simulink model "slrt_parker"  (R2016a)
settings: Solver=FixedStepDiscrete  StartTime=0.0  StopTime=inf  FixedStep=dts  RelTol=1e-3
InitFcn:
  | PARKER_DEPENDENCY
  | Parker_Multi_Axis_Init
  | Parker_ATI_Init
  | Parker_Home_Init
  | Parker_ScopeFormat_Init
undefined symbols (not defined in the file or in its folder): A, accel_filter_coeffs, ATI_torque_Nmm, B, counter_offset, dt, dt_ENC, dts, ENC_obs_filter_coeffs, encoder_counts, F, filter_coeffs_bias, FT_unbias_time, grav_vector, HOMING_dx, HOMING_num_joint, HOMING_tspan, HOMING_Vmov, inv_T, Kd, Kp, N_acceleration, N_bias, N_ENC_obs_filter, N_obs_velocity, N_velocity, pitch, quadrature_mode, R_FT2robot, SafetyMargin, screw_pitch, torque_constant, vel_filter_coeffs, vel_obs_filter_coeffs, Wrench_max
libraries: slrtlib x13, simulink x7, dspswit3 x6, xpcmeasurementcomputinglib x3, xpcconteclib x3, powerlib_meascontrol x2, xpcobsoletelib x1
settings Model: Creator=Roger  LastModifiedBy=arma
settings SolverCC: EnableConcurrentExecution=on
settings DataIOCC: LimitDataPoints=on  SaveFormat=Array  SignalLoggingSaveFormat=ModelDataLogs
settings OptimizationCC: BlockReduction=off  OptimizeBlockIOStorage=off  BufferReuse=off  GlobalBufferReuse=off  ExpressionFolding=off  ExpressionDepthLimit=2147483647  LocalBlockOutputs=off  InitFltsAndDblsToZero=on
settings DebuggingCC: UnderspecifiedInitializationDetection=Classic  MergeDetectMultiDrivingBlocksExec=none  SolverPrmCheckMsg=warning  MultiTaskCondExecSysMsg=warning  MultiTaskRateTransMsg=warning  FcnCallInpInsideContextMsg=EnableAllAsWarning  StateNameClashWarn=warning
settings HardwareCC: ProdBitPerPointer=32  ProdLargestAtomicFloat=None  ProdWordSize=32  ProdLongLongMode=on  ProdHWDeviceType=Generic->32-bit x86 compatible
settings ModelReferenceCC: PropagateSignalLabelsOutOfModel=off
settings SFSimCC: SimParseCustomCode=off
settings RTWCC: SystemTargetFile=slrt.tlc  TemplateMakefile=slrt_default_tmf  Description=Simulink Real-Time  RTWCompilerOptimization=on
settings SimulinkRealTimeCC: GeneratePreprocessorConditionals=Disable all  xPCisDownloadable=off  xPCisModelTimeout=off  xPCModelTimeoutSecs=15
settings ConfigComp: CovModelRefEnable=Off  CovSFcnEnable=off

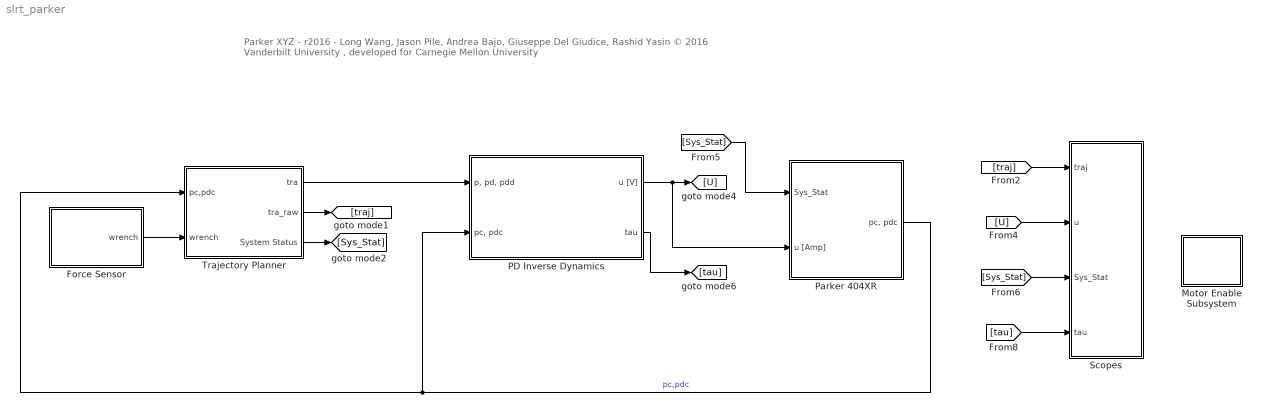
== system slrt_parker ==
  note: Parker XYZ -  r2016 - Long Wang, Jason Pile, Andrea Bajo, Giuseppe Del Giudice, Rashid Yasin
      |  © 2016 Vanderbilt University , developed for Carnegie Mellon University
  Force Sensor : Subsystem
  Motor Enable Subsystem : Subsystem
  PD Inverse Dynamics : Subsystem  TreatAsAtomicUnit=on
  Parker 404XR : Subsystem
  Scopes : Subsystem
  Trajectory Planner : Subsystem  TreatAsAtomicUnit=on
  wires:
  PD Inverse Dynamics/1(u [V]) -> Parker 404XR/2(u [Amp]), [U]
  Parker 404XR/1("pc, pdc") -> Trajectory Planner/1(pc,pdc), PD Inverse Dynamics/2("pc, pdc")  "pc,pdc"
  Trajectory Planner/1(tra) -> PD Inverse Dynamics/1("p, pd, pdd")
  Force Sensor/1(wrench) -> Trajectory Planner/2(wrench)
  [Sys_Stat] -> Parker 404XR/1(Sys_Stat)
  [traj] -> Scopes/1(traj)
  [U] -> Scopes/2(u)
  [Sys_Stat] -> Scopes/3(Sys_Stat)
  PD Inverse Dynamics/2(tau) -> [tau]
  [tau] -> Scopes/4(tau)
  Trajectory Planner/2(tra_raw) -> [traj]
  Trajectory Planner/3(System Status) -> [Sys_Stat]

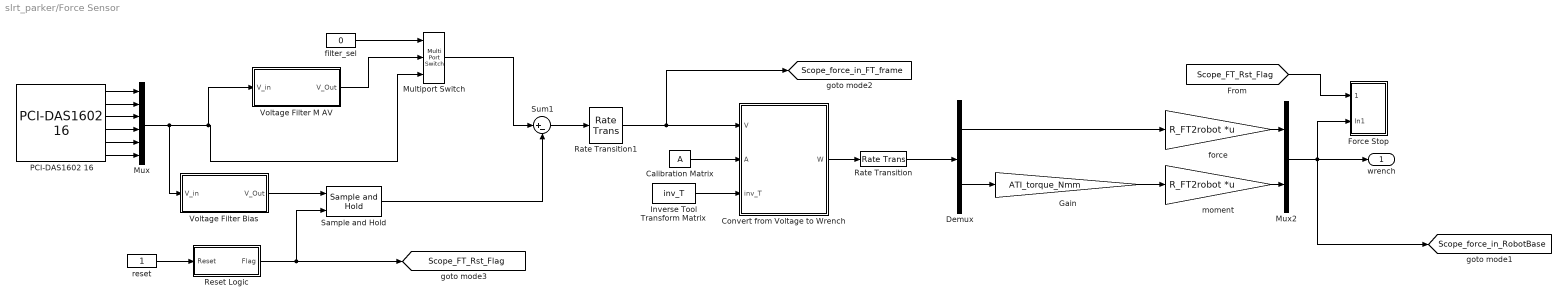
== system slrt_parker/Force Sensor ==
  Calibration Matrix : Constant  Value=A
  Convert from Voltage to Wrench : MATLAB Function  TreatAsAtomicUnit=on
  Demux : Demux  Outputs=2
  Force Stop : Subsystem
  Gain : Gain  Gain=ATI_torque_Nmm
  Inverse Tool Transform Matrix : Constant  Value=inv_T  VectorParams1D=off
  Multiport Switch : MultiPortSwitch  Inputs=2
  Mux : Mux  Inputs=6
  Mux2 : Mux  Inputs=2
  "PCI-DAS1602 16 " : xpcobsoletelib/Measurement Computing obs/A//D/PCI-DAS1602 16   channel=6  range=+-10V  mux=Differential (8 channels)  sampletime=dts  slot=-1
  Rate Transition : RateTransition  OutPortSampleTime=dt
  Rate Transition1 : RateTransition  OutPortSampleTime=dt
  Reset Logic : Subsystem
  Sample and Hold : powerlib_meascontrol/Additional Components/Sample and Hold  ic=zeros(6,1)  Ts=dts
  Sum1 : Sum  Inputs=|+-  SampleTime=dts
  Voltage Filter Bias : Subsystem
  Voltage Filter M AV : Subsystem
  filter_sel : Constant  Value=0
  force : Gain  Gain=R_FT2robot  Multiplication=Matrix(K*u)
  moment : Gain  Gain=R_FT2robot  Multiplication=Matrix(K*u)
  reset : Constant
  wrench : Outport
  tag scope: Scope_FT_Rst_Flag=global, Scope_force_in_FT_frame=global, Scope_force_in_RobotBase=global
  wires:
  "PCI-DAS1602 16 "/1 -> Mux/1
  "PCI-DAS1602 16 "/2 -> Mux/2
  "PCI-DAS1602 16 "/3 -> Mux/3
  "PCI-DAS1602 16 "/4 -> Mux/4
  "PCI-DAS1602 16 "/5 -> Mux/5
  Mux/1 -> Voltage Filter Bias/1(V_in), Voltage Filter M AV/1(V_in), Multiport Switch/3
  "PCI-DAS1602 16 "/6 -> Mux/6
  Calibration Matrix/1 -> Convert from Voltage to Wrench/2(A)
  Inverse Tool Transform Matrix/1 -> Convert from Voltage to Wrench/3(inv_T)
  Sum1/1 -> Rate Transition1/1
  Demux/1 -> force/1
  Demux/2 -> Gain/1
  force/1 -> Mux2/1
  moment/1 -> Mux2/2
  Mux2/1 -> [Scope_force_in_RobotBase], wrench/1, Force Stop/2(In1)
  Convert from Voltage to Wrench/1(W) -> Rate Transition/1
  Rate Transition/1 -> Demux/1
  Multiport Switch/1 -> Sum1/1
  filter_sel/1 -> Multiport Switch/1
  Voltage Filter Bias/1(V_Out) -> Sample and Hold/1
  Sample and Hold/1 -> Sum1/2
  reset/1 -> Reset Logic/1(Reset)
  Reset Logic/1(Flag) -> [Scope_FT_Rst_Flag], Sample and Hold/2
  Rate Transition1/1 -> [Scope_force_in_FT_frame], Convert from Voltage to Wrench/1(V)
  Voltage Filter M AV/1(V_Out) -> Multiport Switch/2
  [Scope_FT_Rst_Flag] -> Force Stop/1(ResetFlag)
  Gain/1 -> moment/1

== system slrt_parker/Motor Enable Subsystem ==
  Demux : Demux  Outputs=3
  Enable Motors : Constant  Value=ones(3,1)
  PCI-DDA08 12 to PORTA : xpcmeasurementcomputinglib/Digital Output/PCI-DDA08 12   channel=[4 5 6]  port=A  reset=[1 1 1]  initValue=[0 0 0]  chip=1  sampletime=dt  slot=-1
  wires:
  Demux/1 -> PCI-DDA08 12 to PORTA/1
  Demux/2 -> PCI-DDA08 12 to PORTA/2
  Demux/3 -> PCI-DDA08 12 to PORTA/3
  Enable Motors/1 -> Demux/1

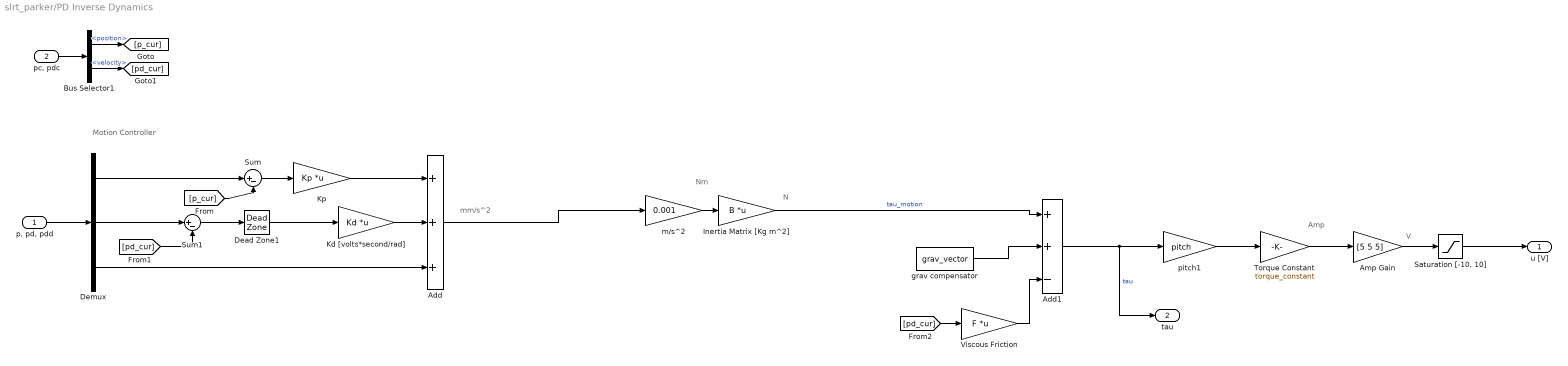
== system slrt_parker/PD Inverse Dynamics ==
  note: Motion Controller
  note: N
  note: mm/s^2
  note: Amp
  note: V
  note: Nm
  "p, pd, pdd" : Inport
  "pc, pdc" : Inport  Port=2
  Add : Sum  Inputs=+++
  Add1 : Sum  Inputs=++-  SampleTime=dt
  Amp Gain : Gain  Gain=[5 5 5]
  Bus Selector1 : BusSelector  OutputSignals=position,velocity
  Dead Zone1 : DeadZone  LowerValue=-2.5  UpperValue=2.5  SaturateOnIntegerOverflow=on
  Demux : Demux  Outputs=[3 3 3]
  Inertia Matrix [Kg m^2] : Gain  Gain=B  Multiplication=Matrix(K*u)
  Kd [volts*second/rad] : Gain  Gain=Kd  Multiplication=Matrix(K*u)
  Kp : Gain  Gain=Kp  Multiplication=Matrix(K*u)
  "Saturation [-10, 10]" : Saturate  UpperLimit=10  LowerLimit=-10
  Sum : Sum  Inputs=|+-
  Sum1 : Sum  Inputs=|+-
  Torque Constant : Gain  Gain=torque_constant
  Viscous Friction : Gain  Gain=F  Multiplication=Matrix(K*u)  SampleTime=dt
  grav compensator : Constant  Value=grav_vector
  m/s^2 : Gain  Gain=0.001
  pitch1 : Gain  Gain=pitch
  u [V] : Outport
  tau : Outport  Port=2
  wires:
  "Saturation [-10, 10]"/1 -> u [V]/1
  m/s^2/1 -> Inertia Matrix [Kg m^2]/1
  Torque Constant/1 -> Amp Gain/1
  Add1/1 -> tau/1, pitch1/1  "tau"
  pitch1/1 -> Torque Constant/1
  Amp Gain/1 -> "Saturation [-10, 10]"/1
  "p, pd, pdd"/1 -> Demux/1
  "pc, pdc"/1 -> Bus Selector1/1
  Sum/1 -> Kp/1
  Demux/1 -> Sum/1
  Demux/2 -> Sum1/1
  Bus Selector1/1 -> [p_cur]  "<position>"
  [p_cur] -> Sum/2
  [pd_cur] -> Sum1/2
  [pd_cur] -> Viscous Friction/1
  Bus Selector1/2 -> [pd_cur]  "<velocity>"
  Kp/1 -> Add/1
  Kd [volts*second/rad]/1 -> Add/2
  Demux/3 -> Add/3
  Add/1 -> m/s^2/1
  Inertia Matrix [Kg m^2]/1 -> Add1/1  "tau_motion"
  grav compensator/1 -> Add1/2
  Sum1/1 -> Dead Zone1/1
  Dead Zone1/1 -> Kd [volts*second/rad]/1
  Viscous Friction/1 -> Add1/3

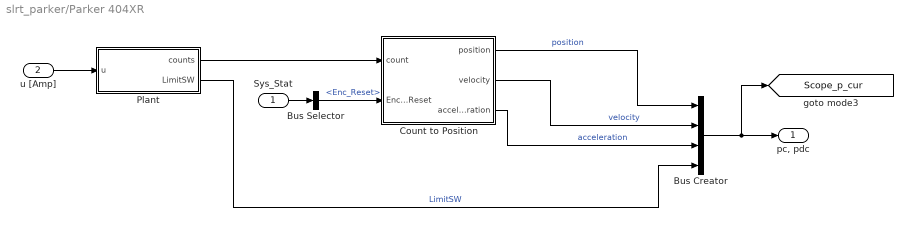
== system slrt_parker/Parker 404XR ==
  Sys_Stat : Inport
  u [Amp] : Inport  Port=2
  Bus Creator : BusCreator  Inputs=4
  Bus Selector : BusSelector  OutputSignals=Enc_Reset
  Count to Position : Subsystem
  Plant : Subsystem
  "pc, pdc" : Outport
  tag scope: Scope_p_cur=global
  wires:
  Count to Position/1(position) -> Bus Creator/1  "position"
  Plant/1(counts) -> Count to Position/1(count)
  u [Amp]/1 -> Plant/1(u)
  Bus Creator/1 -> [Scope_p_cur], "pc, pdc"/1
  Count to Position/2(velocity) -> Bus Creator/2  "velocity"
  Plant/2(LimitSW) -> Bus Creator/4  "LimitSW"
  Sys_Stat/1 -> Bus Selector/1
  Bus Selector/1 -> Count to Position/2(EncoderReset)  "<Enc_Reset>"
  Count to Position/3(acceleration) -> Bus Creator/3  "acceleration"

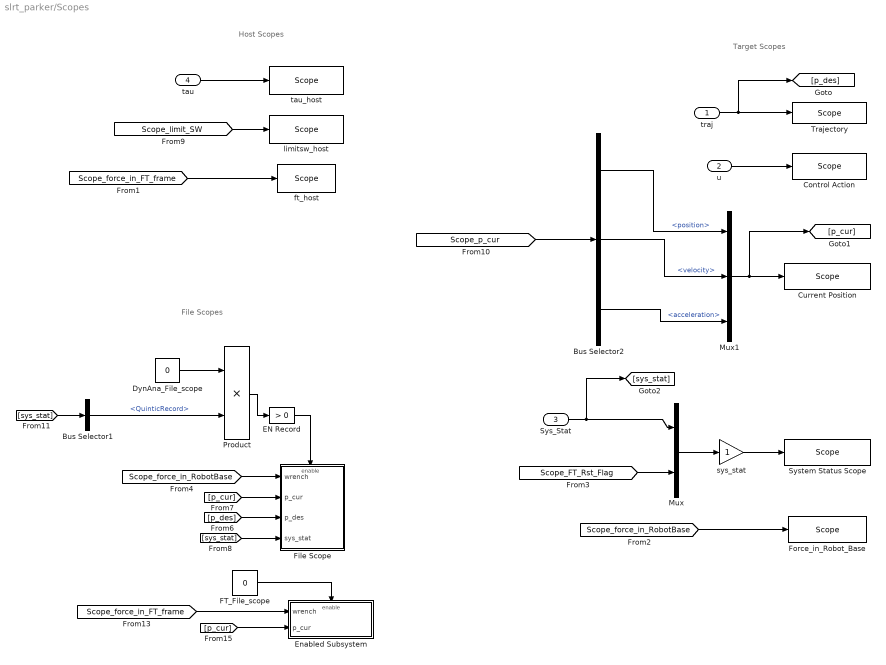
== system slrt_parker/Scopes ==
  note: Host Scopes
  note: File Scopes
  note: Target Scopes
  traj : Inport
  u : Inport  Port=2
  Sys_Stat : Inport  Port=3
  tau : Inport  Port=4
  Bus Selector1 : BusSelector  OutputSignals=QuinticRecord
  Bus Selector2 : BusSelector  OutputSignals=position,velocity,acceleration
  Control Action : slrtlib/Displays and Logging/Scope   scopeno=2  scopetype=Target  autostart=on  viewmode=Numerical  formatstr=Control_Vals_format  grid=on  ylimits=[0,0]  nosamples=Scope_Samples  noprepostsamples=0  interleave=5  triggermode=FreeRun  triggersignal=1  trigsignalfromport=off  triggerlevel=0.0  triggerslope=Either  triggerscope=1  triggersample=0  filename=data.dat  mode=Lazy  writesize=512  autorestart=off  dynamicfilemode=off  maxwritefilesize=512*1024^2
  Current Position : slrtlib/Displays and Logging/Scope   scopeno=3  scopetype=Target  autostart=on  viewmode=Numerical  formatstr=Current_Position_Vals_format  grid=on  ylimits=[0,0]  nosamples=Scope_Samples  noprepostsamples=0  interleave=1  triggermode=FreeRun  triggersignal=1  trigsignalfromport=off  triggerlevel=0.0  triggerslope=Either  triggerscope=1  triggersample=0  filename=data.dat  mode=Lazy  writesize=512  autorestart=off  dynamicfilemode=off  maxwritefilesize=512*1024^2
  DynAna_File_scope : Constant  Value=0
  EN Record : simulink/Logic and Bit Operations/Compare To Constant  relop=>  const=0  OutDataTypeStr=boolean
  Enabled Subsystem : Subsystem  TreatAsAtomicUnit=on
  FT_File_scope : Constant  Value=0
  File Scope : Subsystem
  Force_in_Robot_Base : slrtlib/Displays and Logging/Scope   scopeno=5  scopetype=Target  autostart=on  viewmode=Numerical  formatstr=forceFormat  grid=on  ylimits=[0,0]  nosamples=Scope_Samples  noprepostsamples=0  interleave=1  triggermode=FreeRun  triggersignal=1  trigsignalfromport=off  triggerlevel=0.0  triggerslope=Either  triggerscope=1  triggersample=0  filename=data.dat  mode=Lazy  writesize=512  autorestart=off  dynamicfilemode=off  maxwritefilesize=512*1024^2
  Mux : Mux  Inputs=2
  Mux1 : Mux  Inputs=3
  Product : Product  RndMeth=Zero
  System Status Scope : slrtlib/Displays and Logging/Scope   scopeno=4  scopetype=Target  autostart=on  viewmode=Numerical  formatstr=Scope_format_sys_stat  grid=on  ylimits=[0,0]  nosamples=Scope_Samples  noprepostsamples=0  interleave=1  triggermode=FreeRun  triggersignal=1  trigsignalfromport=off  triggerlevel=0.0  triggerslope=Either  triggerscope=1  triggersample=0  filename=data.dat  mode=Lazy  writesize=512  autorestart=off  dynamicfilemode=off  maxwritefilesize=512*1024^2
  Trajectory : slrtlib/Displays and Logging/Scope   scopeno=1  scopetype=Target  autostart=on  viewmode=Numerical  formatstr=p_cmd_scope_format  grid=on  ylimits=[0,0]  nosamples=25  noprepostsamples=0  interleave=1  triggermode=FreeRun  triggersignal=1  trigsignalfromport=off  triggerlevel=0.0  triggerslope=Either  triggerscope=1  triggersample=0  filename=foamdata1.dat  mode=Lazy  writesize=512  autorestart=off  dynamicfilemode=off  maxwritefilesize=512*1024^2
  ft_host : slrtlib/Displays and Logging/Scope   scopeno=12  scopetype=Host  autostart=on  viewmode=Graphical redraw  formatstr='%15.6f'  grid=on  ylimits=[0,0]  nosamples=Scope_Samples  noprepostsamples=0  interleave=1  triggermode=FreeRun  triggersignal=1  trigsignalfromport=off  triggerlevel=0.0  triggerslope=Either  triggerscope=1  triggersample=0  filename=data.dat  mode=Lazy  writesize=512  autorestart=off  dynamicfilemode=off  maxwritefilesize=512*1024^2
  limitsw_host : slrtlib/Displays and Logging/Scope   scopeno=11  scopetype=Host  autostart=on  viewmode=Graphical redraw  formatstr='%15.6f'  grid=on  ylimits=[0,0]  nosamples=Scope_Samples  noprepostsamples=0  interleave=1  triggermode=FreeRun  triggersignal=1  trigsignalfromport=off  triggerlevel=0.0  triggerslope=Either  triggerscope=1  triggersample=0  filename=data.dat  mode=Lazy  writesize=512  autorestart=off  dynamicfilemode=off  maxwritefilesize=512*1024^2
  sys_stat : Gain
  "tau_host " : slrtlib/Displays and Logging/Scope   scopeno=10  scopetype=Host  autostart=on  viewmode=Graphical redraw  formatstr='%15.6f'  grid=on  ylimits=[0,0]  nosamples=Scope_Samples  noprepostsamples=0  interleave=1  triggermode=FreeRun  triggersignal=1  trigsignalfromport=off  triggerlevel=0.0  triggerslope=Either  triggerscope=1  triggersample=0  filename=data.dat  mode=Lazy  writesize=512  autorestart=off  dynamicfilemode=off  maxwritefilesize=512*1024^2
  wires:
  [Scope_force_in_FT_frame] -> ft_host/1
  [Scope_force_in_RobotBase] -> Force_in_Robot_Base/1
  traj/1 -> [p_des], Trajectory/1
  u/1 -> Control Action/1
  [Scope_limit_SW] -> limitsw_host/1
  Sys_Stat/1 -> Mux/1, [sys_stat]
  tau/1 -> "tau_host "/1
  [Scope_FT_Rst_Flag] -> Mux/2
  Mux/1 -> sys_stat/1
  Mux1/1 -> [p_cur], Current Position/1
  [Scope_force_in_RobotBase] -> File Scope/1(wrench)
  [p_cur] -> File Scope/2(p_cur)
  [p_des] -> File Scope/3(p_des)
  [sys_stat] -> File Scope/4(sys_stat)
  [sys_stat] -> Bus Selector1/1
  EN Record/1 -> File Scope/Enable
  [Scope_p_cur] -> Bus Selector2/1
  Bus Selector2/1 -> Mux1/1  "<position>"
  Bus Selector2/2 -> Mux1/2  "<velocity>"
  Bus Selector2/3 -> Mux1/3  "<acceleration>"
  Bus Selector1/1 -> Product/2  "<QuinticRecord>"
  DynAna_File_scope/1 -> Product/1
  Product/1 -> EN Record/1
  sys_stat/1 -> System Status Scope/1
  [Scope_force_in_FT_frame] -> Enabled Subsystem/1(wrench)
  [p_cur] -> Enabled Subsystem/2(p_cur)
  FT_File_scope/1 -> Enabled Subsystem/Enable

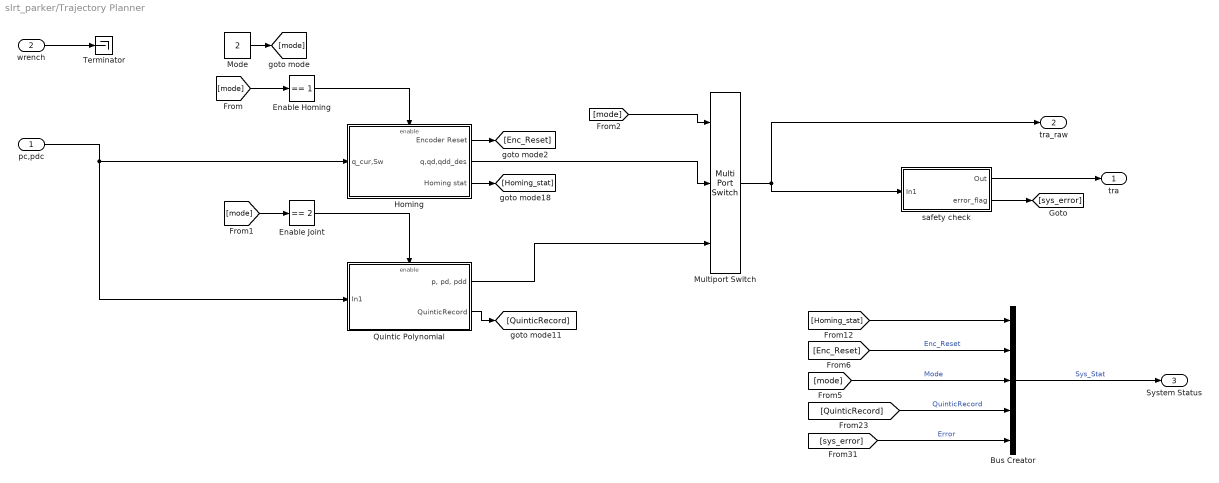
== system slrt_parker/Trajectory Planner ==
  pc,pdc : Inport
  wrench : Inport  Port=2
  Bus Creator : BusCreator  Inputs=5
  Enable Homing : simulink/Logic and Bit Operations/Compare To Constant  relop===  const=1  OutDataTypeStr=boolean
  Enable Joint : simulink/Logic and Bit Operations/Compare To Constant  relop===  const=2  OutDataTypeStr=boolean
  Homing : Subsystem
  Mode : Constant  Value=2
  Multiport Switch : MultiPortSwitch  Inputs=2
  Quintic Polynomial : Subsystem  TreatAsAtomicUnit=on
  Terminator : Terminator
  safety check : Subsystem
  tra : Outport
  tra_raw : Outport  Port=2
  System Status : Outport  Port=3
  wires:
  pc,pdc/1 -> Quintic Polynomial/1(In1), Homing/1(q_cur,Sw)
  Enable Joint/1 -> Quintic Polynomial/Enable
  Homing/2(q,qd,qdd_des) -> Multiport Switch/2
  Quintic Polynomial/1("p, pd, pdd") -> Multiport Switch/3
  Enable Homing/1 -> Homing/Enable
  Mode/1 -> [mode]
  [mode] -> Enable Homing/1
  [mode] -> Enable Joint/1
  [mode] -> Multiport Switch/1
  wrench/1 -> Terminator/1
  Homing/1(Encoder Reset) -> [Enc_Reset]
  Quintic Polynomial/2(QuinticRecord) -> [QuinticRecord]
  Homing/3(Homing stat) -> [Homing_stat]
  Multiport Switch/1 -> tra_raw/1, safety check/1(In1)
  safety check/1(Out) -> tra/1
  safety check/2(error_flag) -> [sys_error]
  Bus Creator/1 -> System Status/1  "Sys_Stat"
  [mode] -> Bus Creator/3  "Mode"
  [Enc_Reset] -> Bus Creator/2  "Enc_Reset"
  [QuinticRecord] -> Bus Creator/4  "QuinticRecord"
  [sys_error] -> Bus Creator/5  "Error"
  [Homing_stat] -> Bus Creator/1

== system slrt_parker/Force Sensor/Force Stop ==
  ResetFlag : Inport
  In1 : Inport  Port=2
  Abs : Abs
  Compare To Constant2 : simulink/Logic and Bit Operations/Compare To Constant  relop=>=  const=SafetyMargin*Wrench_max  OutDataTypeStr=boolean
  Gain : Gain
  MATLAB Function : MATLAB Function  TreatAsAtomicUnit=on
  Product : Product
  Stop Simulation : Stop
  wires:
  Abs/1 -> Gain/1
  Gain/1 -> Compare To Constant2/1
  Compare To Constant2/1 -> Stop Simulation/1
  In1/1 -> Product/1
  Product/1 -> Abs/1
  ResetFlag/1 -> MATLAB Function/1(u)
  MATLAB Function/1(y) -> Product/2

== system slrt_parker/Force Sensor/Reset Logic ==
  Reset : Inport
  Const1 : Constant
  Const2 : Constant  Value=0
  Const3 : Constant  Value=0
  N-Sample Switch : dspswit3/N-Sample Switch  N=FT_unbias_time/dts  reset=on  TriggerType=Rising edge  Ts=dts
  N-Sample Switch1 : dspswit3/N-Sample Switch  N=1  reset=off  TriggerType=Rising edge  Ts=dts
  Flag : Outport
  wires:
  Const1/1 -> N-Sample Switch/1
  N-Sample Switch/1 -> Flag/1
  Const2/1 -> N-Sample Switch/2
  Reset/1 -> N-Sample Switch1/2
  N-Sample Switch1/1 -> N-Sample Switch/3
  Const3/1 -> N-Sample Switch1/1

== system slrt_parker/Force Sensor/Voltage Filter Bias ==
  V_in : Inport  SampleTime=dts
  Discrete FIR Filter : DiscreteFir  CoefSource=Input port  SampleTime=dts  AccumDataTypeStr=Inherit: Same as product output
      settings: InputPortMap=u0,u1
  Gain : Gain  Gain=1/N_bias  SampleTime=dts
  filter_coeffs : Constant  Value=filter_coeffs_bias  SampleTime=dts
  V_Out : Outport  SampleTime=dts
  wires:
  Gain/1 -> V_Out/1
  filter_coeffs/1 -> Discrete FIR Filter/2
  Discrete FIR Filter/1 -> Gain/1
  V_in/1 -> Discrete FIR Filter/1

== system slrt_parker/Force Sensor/Voltage Filter M AV ==
  V_in : Inport  SampleTime=dts
  Discrete FIR Filter : DiscreteFir  CoefSource=Input port  SampleTime=dts  AccumDataTypeStr=Inherit: Same as product output
      settings: InputPortMap=u0,u1
  Gain : Gain  Gain=1/(dt/dts)  SampleTime=dts
  filter_coeffs : Constant  Value=ones(dt/dts,1)  SampleTime=dts
  V_Out : Outport  SampleTime=dts
  wires:
  V_in/1 -> Discrete FIR Filter/1
  Discrete FIR Filter/1 -> Gain/1
  filter_coeffs/1 -> Discrete FIR Filter/2
  Gain/1 -> V_Out/1

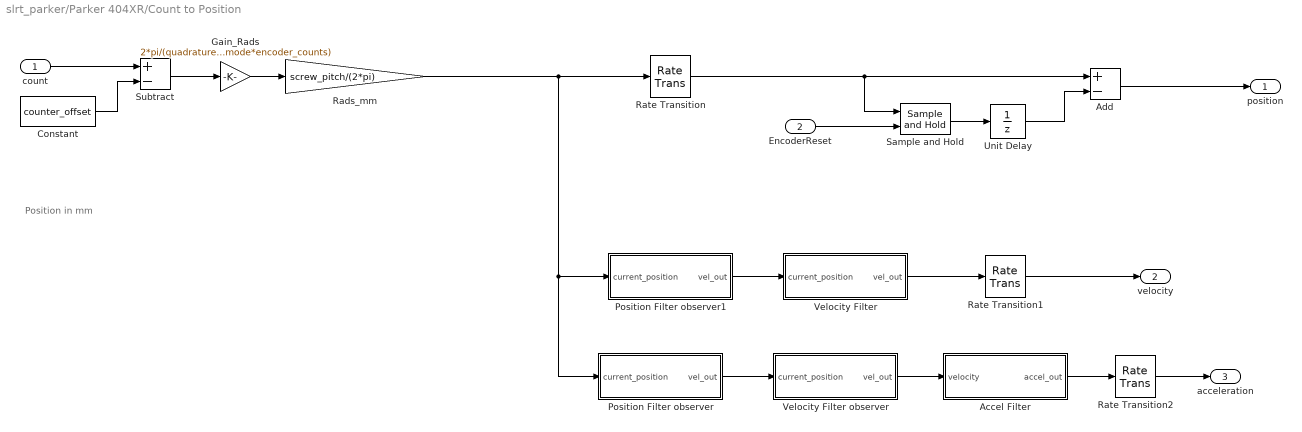
== system slrt_parker/Parker 404XR/Count to Position ==
  note: Position in mm
  count : Inport
  EncoderReset : Inport  Port=2
  Accel Filter : Subsystem
  Add : Sum  Inputs=+-
  Constant : Constant  Value=counter_offset
  Gain_Rads : Gain  Gain=2*pi/(quadrature_mode*encoder_counts)
  Position Filter observer : Subsystem
  Position Filter observer1 : Subsystem
  Rads_mm : Gain  Gain=screw_pitch/(2*pi)
  Rate Transition : RateTransition  OutPortSampleTime=dt
  Rate Transition1 : RateTransition  OutPortSampleTime=dt
  Rate Transition2 : RateTransition  OutPortSampleTime=dt
  Sample and Hold : powerlib_meascontrol/Additional Components/Sample and Hold  ic=zeros(3,1)  Ts=dt
  Subtract : Sum  Inputs=+-
  Unit Delay : UnitDelay  SampleTime=-1
  Velocity Filter : Subsystem
  Velocity Filter observer : Subsystem
  position : Outport
  velocity : Outport  Port=2
  acceleration : Outport  Port=3
  wires:
  Constant/1 -> Subtract/2
  count/1 -> Subtract/1
  Subtract/1 -> Gain_Rads/1
  Gain_Rads/1 -> Rads_mm/1
  Add/1 -> position/1
  Rads_mm/1 -> Rate Transition/1, Position Filter observer1/1(current_position), Position Filter observer/1(current_position)
  Velocity Filter/1(vel_out) -> Rate Transition1/1
  Accel Filter/1(accel_out) -> Rate Transition2/1
  Velocity Filter observer/1(vel_out) -> Accel Filter/1(velocity)
  Position Filter observer/1(vel_out) -> Velocity Filter observer/1(current_position)
  Position Filter observer1/1(vel_out) -> Velocity Filter/1(current_position)
  Sample and Hold/1 -> Unit Delay/1
  Rate Transition/1 -> Sample and Hold/1, Add/1
  Rate Transition1/1 -> velocity/1
  Rate Transition2/1 -> acceleration/1
  EncoderReset/1 -> Sample and Hold/2
  Unit Delay/1 -> Add/2

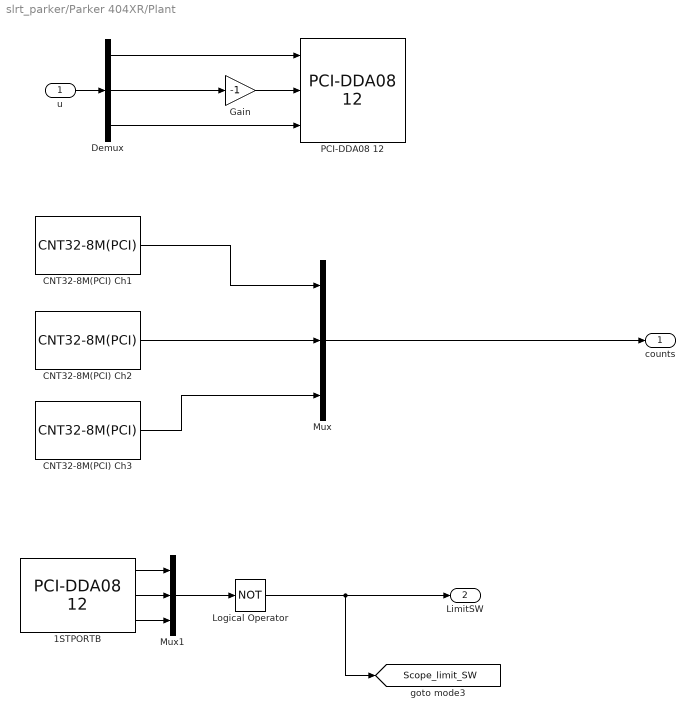
== system slrt_parker/Parker 404XR/Plant ==
  u : Inport
  "1STPORTB " : xpcmeasurementcomputinglib/Digital Input/PCI-DDA08 12   channel=[3 4 7]  port=C  chip=1  sampletime=dt  slot=-1
  CNT32-8M(PCI) Ch1 : xpcconteclib/Incremental Encoder/CNT32-8M(PCI)   Channel=1  OperationMode=2-phase Input Synchronous Clear Multiply by 4  DigitalFilter=No filtering  PulseInput=Differential line receiver input  Direction=Down in the clockwise direction/Up in the counterclockwise direction  InitialValue=counter_offset  LoadInitialValue=on  SampleTime=dt_ENC  PciSlot=-1  StartMethod=Model Start  StopMethod=Model Terminate  ZeroClearRising=off  ZeroClearFalling=off  ZeroClearMatch0=off  ZeroClearMatch1=off  PresetRising=off  PresetFalling=off  PresetMatch0=off  PresetMatch1=off  PresetValue=0  Match0Value=0  Match1Value=0  OutputSignalMatch0=off  OutputSignalMatch1=off  OutputSignalAbnormal=off  OutputSignalDigitalFilter=off  OutputSignalAlarm=off  OneShotDuration=10 microseconds  IndexEnable=Disable  IndexLogic=Positive (Active High)  EnableDigitalInput=off  EnableDigitalOutput=off  DigitalOutputInitialValue=None  DigitalOutputFinalValue=None
  CNT32-8M(PCI) Ch2 : xpcconteclib/Incremental Encoder/CNT32-8M(PCI)   Channel=2  OperationMode=2-phase Input Synchronous Clear Multiply by 4  DigitalFilter=No filtering  PulseInput=Differential line receiver input  Direction=Up in the clockwise direction/Down in the counterclockwise direction  InitialValue=counter_offset  LoadInitialValue=on  SampleTime=dt_ENC  PciSlot=-1  StartMethod=Model Start  StopMethod=Model Terminate  ZeroClearRising=off  ZeroClearFalling=off  ZeroClearMatch0=off  ZeroClearMatch1=off  PresetRising=off  PresetFalling=off  PresetMatch0=off  PresetMatch1=off  PresetValue=0  Match0Value=0  Match1Value=0  OutputSignalMatch0=off  OutputSignalMatch1=off  OutputSignalAbnormal=off  OutputSignalDigitalFilter=off  OutputSignalAlarm=off  OneShotDuration=10 microseconds  IndexEnable=Disable  IndexLogic=Positive (Active High)  EnableDigitalInput=off  EnableDigitalOutput=off  DigitalOutputInitialValue=None  DigitalOutputFinalValue=None
  CNT32-8M(PCI) Ch3 : xpcconteclib/Incremental Encoder/CNT32-8M(PCI)   Channel=3  OperationMode=2-phase Input Synchronous Clear Multiply by 4  DigitalFilter=No filtering  PulseInput=Differential line receiver input  Direction=Down in the clockwise direction/Up in the counterclockwise direction  InitialValue=counter_offset  LoadInitialValue=on  SampleTime=dt_ENC  PciSlot=-1  StartMethod=Model Start  StopMethod=Model Terminate  ZeroClearRising=off  ZeroClearFalling=off  ZeroClearMatch0=off  ZeroClearMatch1=off  PresetRising=off  PresetFalling=off  PresetMatch0=off  PresetMatch1=off  PresetValue=0  Match0Value=0  Match1Value=0  OutputSignalMatch0=off  OutputSignalMatch1=off  OutputSignalAbnormal=off  OutputSignalDigitalFilter=off  OutputSignalAlarm=off  OneShotDuration=10 microseconds  IndexEnable=Disable  IndexLogic=Positive (Active High)  EnableDigitalInput=off  EnableDigitalOutput=off  DigitalOutputInitialValue=None  DigitalOutputFinalValue=None
  Demux : Demux  Outputs=3
  Gain : Gain  Gain=-1
  Logical Operator : Logic  Operator=NOT  Inputs=1  AllPortsSameDT=off  OutDataTypeStr=boolean
  Mux : Mux  Inputs=3
  Mux1 : Mux  Inputs=3
  "PCI-DDA08 12 " : xpcmeasurementcomputinglib/D//A/PCI-DDA08 12   channel=[4 5 6]  range=[-10 -10 -10]  reset=[1 1 1]  initValue=[0 0 0]  sampletime=dt  pci_dev=-1
  counts : Outport
  LimitSW : Outport  Port=2
  tag scope: Scope_limit_SW=global
  wires:
  Demux/3 -> "PCI-DDA08 12 "/3
  Gain/1 -> "PCI-DDA08 12 "/2
  CNT32-8M(PCI) Ch3/1 -> Mux/3
  CNT32-8M(PCI) Ch2/1 -> Mux/2
  CNT32-8M(PCI) Ch1/1 -> Mux/1
  Demux/2 -> Gain/1
  Demux/1 -> "PCI-DDA08 12 "/1
  u/1 -> Demux/1
  "1STPORTB "/1 -> Mux1/1
  "1STPORTB "/2 -> Mux1/2
  "1STPORTB "/3 -> Mux1/3
  Mux/1 -> counts/1
  Mux1/1 -> Logical Operator/1
  Logical Operator/1 -> [Scope_limit_SW], LimitSW/1

== system slrt_parker/Scopes/Enabled Subsystem ==
  wrench : Inport
  p_cur : Inport  Port=2
  Enable : EnablePort
  Gain : Gain
  Gain1 : Gain
  "ft_Scope " : slrtlib/Displays and Logging/Scope   scopeno=23  scopetype=File  autostart=on  viewmode=Graphical redraw  formatstr='%15.6f'  grid=on  ylimits=[0,0]  nosamples=50000  noprepostsamples=0  interleave=1  triggermode=FreeRun  triggersignal=1  trigsignalfromport=off  triggerlevel=0.0  triggerslope=Either  triggerscope=1  triggersample=0  filename=Ft_<%%%>.dat  mode=Lazy  writesize=512  autorestart=on  dynamicfilemode=on  maxwritefilesize=512*1024^2
  "pc_Scope " : slrtlib/Displays and Logging/Scope   scopeno=24  scopetype=File  autostart=on  viewmode=Graphical redraw  formatstr='%15.6f'  grid=on  ylimits=[0,0]  nosamples=50000  noprepostsamples=0  interleave=1  triggermode=FreeRun  triggersignal=1  trigsignalfromport=off  triggerlevel=0.0  triggerslope=Either  triggerscope=1  triggersample=0  filename=Pc_<%%%>.dat  mode=Lazy  writesize=512  autorestart=on  dynamicfilemode=on  maxwritefilesize=512*1024^2
  wires:
  wrench/1 -> Gain1/1
  p_cur/1 -> Gain/1
  Gain/1 -> "pc_Scope "/1
  Gain1/1 -> "ft_Scope "/1

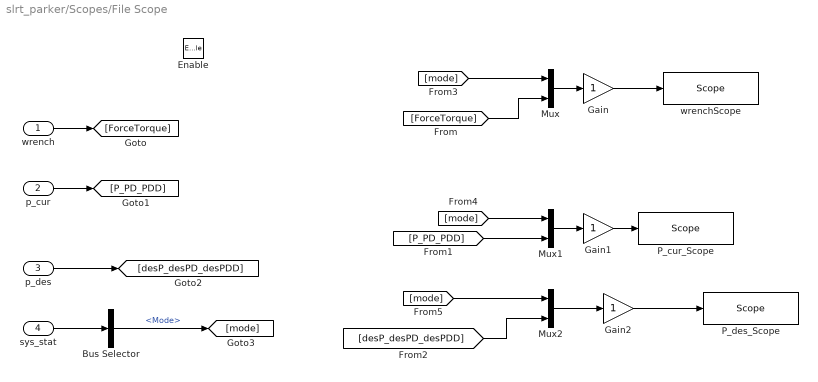
== system slrt_parker/Scopes/File Scope ==
  wrench : Inport
  p_cur : Inport  Port=2
  p_des : Inport  Port=3
  sys_stat : Inport  Port=4
  Enable : EnablePort
  Bus Selector : BusSelector  OutputSignals=Mode
  Gain : Gain
  Gain1 : Gain
  Gain2 : Gain
  Mux : Mux  Inputs=2
  Mux1 : Mux  Inputs=2
  Mux2 : Mux  Inputs=2
  P_cur_Scope : slrtlib/Displays and Logging/Scope   scopeno=21  scopetype=File  autostart=on  viewmode=Numerical  formatstr=forceFormat  grid=on  ylimits=[0,0]  nosamples=50000  noprepostsamples=0  interleave=1  triggermode=FreeRun  triggersignal=1  trigsignalfromport=off  triggerlevel=0.0  triggerslope=Either  triggerscope=1  triggersample=0  filename=Cur_<%%%>.dat  mode=Lazy  writesize=512  autorestart=on  dynamicfilemode=on  maxwritefilesize=512*1024^2
  P_des_Scope : slrtlib/Displays and Logging/Scope   scopeno=22  scopetype=File  autostart=on  viewmode=Numerical  formatstr=forceFormat  grid=on  ylimits=[0,0]  nosamples=50000  noprepostsamples=0  interleave=1  triggermode=FreeRun  triggersignal=1  trigsignalfromport=off  triggerlevel=0.0  triggerslope=Either  triggerscope=1  triggersample=0  filename=Des_<%%%>.dat  mode=Lazy  writesize=512  autorestart=on  dynamicfilemode=on  maxwritefilesize=512*1024^2
  wrenchScope : slrtlib/Displays and Logging/Scope   scopeno=20  scopetype=File  autostart=on  viewmode=Numerical  formatstr=forceFormat  grid=on  ylimits=[0,0]  nosamples=50000  noprepostsamples=0  interleave=1  triggermode=FreeRun  triggersignal=1  trigsignalfromport=off  triggerlevel=0.0  triggerslope=Either  triggerscope=1  triggersample=0  filename=We_<%%%>.dat  mode=Lazy  writesize=512  autorestart=on  dynamicfilemode=on  maxwritefilesize=512*1024^2
  wires:
  wrench/1 -> [ForceTorque]
  p_cur/1 -> [P_PD_PDD]
  p_des/1 -> [desP_desPD_desPDD]
  sys_stat/1 -> Bus Selector/1
  Bus Selector/1 -> [mode]  "<Mode>"
  Mux/1 -> Gain/1
  [ForceTorque] -> Mux/2
  [mode] -> Mux/1
  Mux1/1 -> Gain1/1
  [mode] -> Mux1/1
  [P_PD_PDD] -> Mux1/2
  Mux2/1 -> Gain2/1
  [mode] -> Mux2/1
  [desP_desPD_desPDD] -> Mux2/2
  Gain/1 -> wrenchScope/1
  Gain1/1 -> P_cur_Scope/1
  Gain2/1 -> P_des_Scope/1

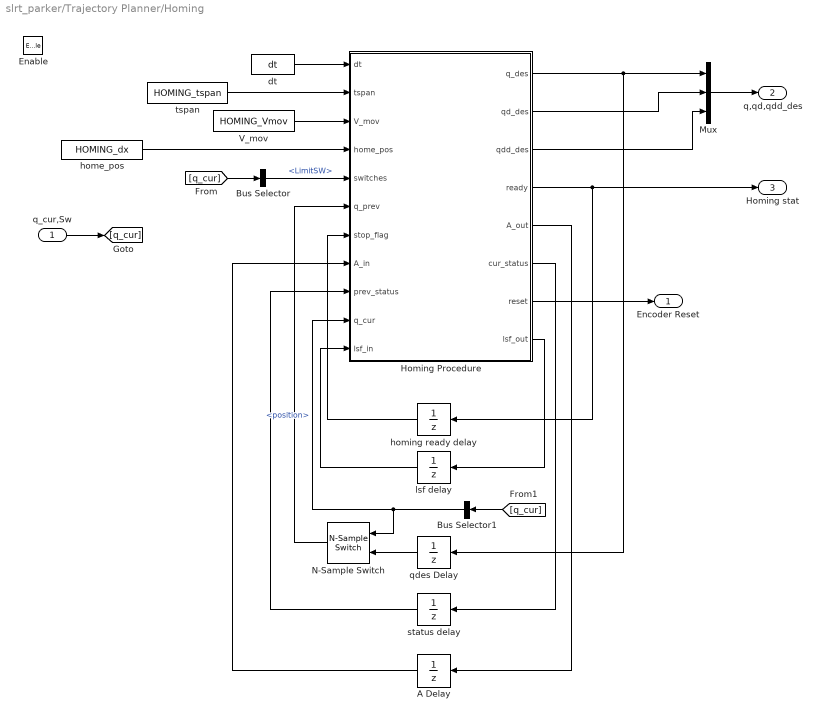
== system slrt_parker/Trajectory Planner/Homing ==
  q_cur,Sw : Inport
  Enable : EnablePort  StatesWhenEnabling=reset
  A Delay : UnitDelay  InitialCondition=zeros(HOMING_num_joint,4)  SampleTime=dt
  Bus Selector : BusSelector  OutputSignals=LimitSW
  Bus Selector1 : BusSelector  OutputSignals=position
  Homing Procedure : MATLAB Function  TreatAsAtomicUnit=on
  Mux : Mux  Inputs=3
  N-Sample Switch : dspswit3/N-Sample Switch  N=1  reset=off  TriggerType=Rising edge  Ts=dt
  V_mov : Constant  Value=HOMING_Vmov  SampleTime=dt
  dt : Constant  Value=dt  SampleTime=dt
  home_pos : Constant  Value=HOMING_dx  SampleTime=dt
  homing ready delay : UnitDelay  SampleTime=dt
  lsf delay : UnitDelay  InitialCondition=ones(HOMING_num_joint,1)  SampleTime=dt
  qdes Delay : UnitDelay  InitialCondition=zeros(HOMING_num_joint,1)  SampleTime=dt
  status delay : UnitDelay  SampleTime=dt
  tspan : Constant  Value=HOMING_tspan  SampleTime=dt
  Encoder Reset : Outport
  q,qd,qdd_des : Outport  Port=2
  Homing stat : Outport  Port=3
  wires:
  Homing Procedure/1(q_des) -> qdes Delay/1, Mux/1
  Bus Selector/1 -> Homing Procedure/5(switches)  "<LimitSW>"
  Homing Procedure/4(ready) -> homing ready delay/1, Homing stat/1
  homing ready delay/1 -> Homing Procedure/7(stop_flag)
  dt/1 -> Homing Procedure/1(dt)
  qdes Delay/1 -> N-Sample Switch/2
  N-Sample Switch/1 -> Homing Procedure/6(q_prev)
  Bus Selector1/1 -> Homing Procedure/10(q_cur), N-Sample Switch/1  "<position>"
  home_pos/1 -> Homing Procedure/4(home_pos)
  Homing Procedure/5(A_out) -> A Delay/1
  A Delay/1 -> Homing Procedure/8(A_in)
  Homing Procedure/6(cur_status) -> status delay/1
  status delay/1 -> Homing Procedure/9(prev_status)
  Homing Procedure/7(reset) -> Encoder Reset/1
  Homing Procedure/8(lsf_out) -> lsf delay/1
  lsf delay/1 -> Homing Procedure/11(lsf_in)
  Homing Procedure/2(qd_des) -> Mux/2
  Homing Procedure/3(qdd_des) -> Mux/3
  Mux/1 -> q,qd,qdd_des/1
  q_cur,Sw/1 -> [q_cur]
  [q_cur] -> Bus Selector/1
  [q_cur] -> Bus Selector1/1
  tspan/1 -> Homing Procedure/2(tspan)
  V_mov/1 -> Homing Procedure/3(V_mov)

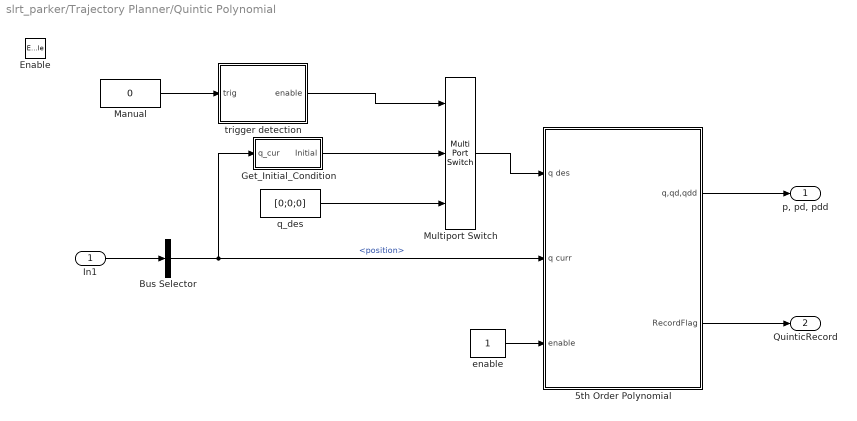
== system slrt_parker/Trajectory Planner/Quintic Polynomial ==
  In1 : Inport
  Enable : EnablePort  StatesWhenEnabling=reset
  5th Order Polynomial : Subsystem
  Bus Selector : BusSelector  OutputSignals=position
  Get_Initial_Condition : Subsystem
  Manual : Constant  Value=0
  Multiport Switch : MultiPortSwitch  DataPortOrder=Zero-based contiguous  Inputs=2
  enable : Constant
  q_des : Constant  Value=[0;0;0]
  trigger detection : Subsystem
  "p, pd, pdd" : Outport  InitialOutput=zeros(9,1)
  QuinticRecord : Outport  Port=2  InitialOutput=0
  wires:
  enable/1 -> 5th Order Polynomial/3(enable)
  In1/1 -> Bus Selector/1
  Bus Selector/1 -> 5th Order Polynomial/2(q curr), Get_Initial_Condition/1(q_cur)  "<position>"
  5th Order Polynomial/1(q,qd,qdd) -> "p, pd, pdd"/1
  Multiport Switch/1 -> 5th Order Polynomial/1(q des)
  q_des/1 -> Multiport Switch/3
  Get_Initial_Condition/1(Initial) -> Multiport Switch/2
  5th Order Polynomial/2(RecordFlag) -> QuinticRecord/1
  Manual/1 -> trigger detection/1(trig)
  trigger detection/1(enable) -> Multiport Switch/1

== system slrt_parker/Trajectory Planner/safety check ==
  In1 : Inport
  Unit Delay2 : UnitDelay  InitialCondition=zeros(9,1)  SampleTime=-1
  Unit Delay3 : UnitDelay  SampleTime=-1
  false detection : MATLAB Function  TreatAsAtomicUnit=on
  Out : Outport
  error_flag : Outport  Port=2
  wires:
  false detection/1(pva_allowed) -> Unit Delay2/1, Out/1
  Unit Delay2/1 -> false detection/2(pva_prev)
  In1/1 -> false detection/1(pva_cmd)
  Unit Delay3/1 -> false detection/3(error_prev)
  false detection/2(error_flag) -> Unit Delay3/1, error_flag/1

== system slrt_parker/Parker 404XR/Count to Position/Accel Filter ==
  note: current velocity
  velocity : Inport
  Discrete Derivative1 : simulink/Discrete/Discrete Derivative  gainval=1.0  ICPrevScaledInput=0.0  InputProcessing=Inherited  OutMin=[]  OutMax=[]  OutDataType=sfix(16)  OutScaling=2^-10  DoSatur=off
  Discrete FIR Filter : DiscreteFir  CoefSource=Input port  AccumDataTypeStr=Inherit: Same as product output
      settings: InputPortMap=u0,u1
  Gain : Gain  Gain=1/N_acceleration
  vel_filter_coeffs : Constant  Value=accel_filter_coeffs
  accel_out : Outport
  wires:
  Discrete FIR Filter/1 -> Gain/1
  vel_filter_coeffs/1 -> Discrete FIR Filter/2
  Gain/1 -> accel_out/1
  velocity/1 -> Discrete Derivative1/1
  Discrete Derivative1/1 -> Discrete FIR Filter/1

== system slrt_parker/Parker 404XR/Count to Position/Position Filter observer ==
  note: current velocity
  current_position : Inport
  Discrete FIR Filter : DiscreteFir  CoefSource=Input port  AccumDataTypeStr=Inherit: Same as product output
      settings: InputPortMap=u0,u1
  Gain : Gain  Gain=1/N_ENC_obs_filter
  encoder obsever filter : Constant  Value=ENC_obs_filter_coeffs
  vel_out : Outport
  wires:
  current_position/1 -> Discrete FIR Filter/1
  Gain/1 -> vel_out/1
  encoder obsever filter/1 -> Discrete FIR Filter/2
  Discrete FIR Filter/1 -> Gain/1

== system slrt_parker/Parker 404XR/Count to Position/Position Filter observer1 ==
  note: current velocity
  current_position : Inport
  Discrete FIR Filter : DiscreteFir  CoefSource=Input port  AccumDataTypeStr=Inherit: Same as product output
      settings: InputPortMap=u0,u1
  Gain : Gain  Gain=1/N_ENC_obs_filter
  encoder obsever filter : Constant  Value=ENC_obs_filter_coeffs
  vel_out : Outport
  wires:
  Discrete FIR Filter/1 -> Gain/1
  encoder obsever filter/1 -> Discrete FIR Filter/2
  Gain/1 -> vel_out/1
  current_position/1 -> Discrete FIR Filter/1

== system slrt_parker/Parker 404XR/Count to Position/Velocity Filter ==
  note: current velocity
  current_position : Inport
  Discrete Derivative : simulink/Discrete/Discrete Derivative  gainval=1.0  ICPrevScaledInput=0.0  InputProcessing=Inherited  OutMin=[]  OutMax=[]  OutDataType=sfix(16)  OutScaling=2^-10  DoSatur=off
  Discrete FIR Filter : DiscreteFir  CoefSource=Input port  AccumDataTypeStr=Inherit: Same as product output
      settings: InputPortMap=u0,u1
  Gain : Gain  Gain=1/N_velocity
  vel_filter_coeffs : Constant  Value=vel_filter_coeffs
  vel_out : Outport
  wires:
  current_position/1 -> Discrete Derivative/1
  Discrete Derivative/1 -> Discrete FIR Filter/1
  Gain/1 -> vel_out/1
  vel_filter_coeffs/1 -> Discrete FIR Filter/2
  Discrete FIR Filter/1 -> Gain/1

== system slrt_parker/Parker 404XR/Count to Position/Velocity Filter observer ==
  note: current velocity
  current_position : Inport
  Discrete Derivative : simulink/Discrete/Discrete Derivative  gainval=1.0  ICPrevScaledInput=0.0  InputProcessing=Inherited  OutMin=[]  OutMax=[]  OutDataType=sfix(16)  OutScaling=2^-10  DoSatur=off
  Discrete FIR Filter : DiscreteFir  CoefSource=Input port  AccumDataTypeStr=Inherit: Same as product output
      settings: InputPortMap=u0,u1
  Gain : Gain  Gain=1/N_obs_velocity
  vel_filter_coeffs : Constant  Value=vel_obs_filter_coeffs
  vel_out : Outport
  wires:
  Discrete FIR Filter/1 -> Gain/1
  vel_filter_coeffs/1 -> Discrete FIR Filter/2
  Gain/1 -> vel_out/1
  Discrete Derivative/1 -> Discrete FIR Filter/1
  current_position/1 -> Discrete Derivative/1

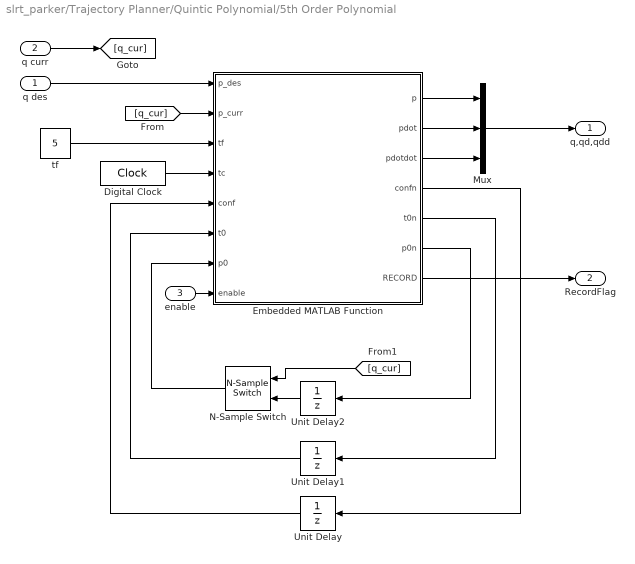
== system slrt_parker/Trajectory Planner/Quintic Polynomial/5th Order Polynomial ==
  q des : Inport
  q curr : Inport  Port=2
  enable : Inport  Port=3
  Digital Clock : DigitalClock  SampleTime=dt
  Embedded MATLAB Function : MATLAB Function  TreatAsAtomicUnit=on
  Mux : Mux  Inputs=3
  N-Sample Switch : dspswit3/N-Sample Switch  N=1  reset=off  TriggerType=Rising edge  Ts=dt
  Unit Delay : UnitDelay  SampleTime=dt
  Unit Delay1 : UnitDelay  SampleTime=dt
  Unit Delay2 : UnitDelay  SampleTime=dt
  tf : Constant  Value=5  SampleTime=dt
  q,qd,qdd : Outport
  RecordFlag : Outport  Port=2
  wires:
  Embedded MATLAB Function/4(confn) -> Unit Delay/1
  Unit Delay/1 -> Embedded MATLAB Function/5(conf)
  Embedded MATLAB Function/5(t0n) -> Unit Delay1/1
  Embedded MATLAB Function/6(p0n) -> Unit Delay2/1
  Unit Delay1/1 -> Embedded MATLAB Function/6(t0)
  Digital Clock/1 -> Embedded MATLAB Function/4(tc)
  q des/1 -> Embedded MATLAB Function/1(p_des)
  tf/1 -> Embedded MATLAB Function/3(tf)
  enable/1 -> Embedded MATLAB Function/8(enable)
  Embedded MATLAB Function/1(p) -> Mux/1
  Embedded MATLAB Function/2(pdot) -> Mux/2
  Mux/1 -> q,qd,qdd/1
  Embedded MATLAB Function/3(pdotdot) -> Mux/3
  N-Sample Switch/1 -> Embedded MATLAB Function/7(p0)
  Unit Delay2/1 -> N-Sample Switch/2
  q curr/1 -> [q_cur]
  [q_cur] -> Embedded MATLAB Function/2(p_curr)
  [q_cur] -> N-Sample Switch/1
  Embedded MATLAB Function/7(RECORD) -> RecordFlag/1

== system slrt_parker/Trajectory Planner/Quintic Polynomial/Get_Initial_Condition ==
  q_cur : Inport
  N-Sample Switch : dspswit3/N-Sample Switch  N=1  reset=off  TriggerType=Rising edge  Ts=dt
  Unit Delay : UnitDelay  InitialCondition=zeros(3,1)  SampleTime=-1
  Initial : Outport
  wires:
  N-Sample Switch/1 -> Unit Delay/1, Initial/1
  Unit Delay/1 -> N-Sample Switch/2
  q_cur/1 -> N-Sample Switch/1

== system slrt_parker/Trajectory Planner/Quintic Polynomial/trigger detection ==
  trig : Inport
  Counter : dspswit3/Counter  Direction=Up  CountEvent=Rising edge  CounterSize=User defined  MaxCount=255  InitialCount=0  Output=Count  HitValue=32  ResetInput=off  SamplesPerFrame=1  Ts=1  CntDtype=double  HitDtype=Boolean
  MATLAB Function : MATLAB Function  TreatAsAtomicUnit=on
  Unit Delay : UnitDelay  SampleTime=dt
  enable : Outport
  wires:
  MATLAB Function/1(enable) -> enable/1, Unit Delay/1
  Counter/1 -> MATLAB Function/1(trig)
  Unit Delay/1 -> MATLAB Function/2(trig_history)
  trig/1 -> Counter/1

== matlab function slrt_parker/Trajectory Planner/Homing/Homing Procedure ==
  data: dt input; tspan input; V_mov input; home_pos input; switches input; q_prev input; q_des output; qd_des output; qdd_des output; ready output; stop_flag input; A_in input; prev_status input; A_out output; cur_status output; reset output; q_cur input; lsf_in input; lsf_out output
% this function executes a homing sequence for the parallel robots
% status definition:
%       1: keep homing
%       0: stop homing
% stop flag definition:
%       0: all limit switches have not been reached
%       1: limit switches reached, calculate trajectory to home config
%       2: run 5th order poly
%       3: home complete - reset and hold position
%       4: turn off reset, hold at 0

function [q_des,qd_des,qdd_des,ready,A_out,cur_status,reset,lsf_out] = homing(dt,tspan,V_mov,home_pos,switches,q_prev,stop_flag,A_in,prev_status,q_cur,lsf_in)
% V_mov=5; % leg velocity while homing (mm/s)
% tspan=10;    % time to execute path plan (sec)
N=length(q_prev);
qd_des=zeros(N,1); % default desired velocity
qdd_des=zeros(N,1); %default desired acceleration

% read limit switches
% when limit switches are reached, switch=1
status=ones(N,1)-switches;    % update triggered switches
lsf_out=lsf_in.*status;
if stop_flag==1
    dx=home_pos;    % total displacement
    A_out=zeros(N,4);   % allocate memory for coefficients

    % construct coefficients
    for i=1:N
        A_out(i,:)=[q_prev(i),10*dx(i), -15*dx(i), 6*dx(i)];
    end
    cur_status=1;
    cur_t=cur_status*dt/tspan;
    T=[1;cur_t^3;cur_t^4;cur_t^5];    % exponential time vector
    q_des=A_out*T;  % current desired position 
    ready=2;        % continue with path plan (should be 2)
    reset=0;
elseif stop_flag==2
    
    if prev_status>=(tspan/dt)    % reached position goal
        T=[1;1;1;1];
        q_des=A_in*T;
        cur_status=prev_status;
        A_out=[q_des,zeros(N,3)];
        ready=3;
        reset=0;
    else    % continue on the trajectory
        cur_t=prev_status*dt/tspan; % current normalized time [0 -> 1]
        T=[1;cur_t^3;cur_t^4;cur_t^5];    % exponential time vector
        q_des=A_in*T;  % current desired position
        cur_status=prev_status+1; % update status step
        A_out=A_in; % maintain current coefficients  
        ready=2;
        reset=0;
    end
elseif stop_flag==3
    cur_status=0;
    A_out=zeros(N,4);
    q_des=q_cur;
    ready=4;
    reset=1;
elseif stop_flag==4
    cur_status=0;
    A_out=zeros(N,4);
    q_des=q_cur*0;
    ready=4;
    reset=0;
else
    % check homing status    
    if (sum(lsf_out))==0   % all limit switches have been reached
        q_des=q_prev;       % stop motion
        ready=1;            % homing finished
        cur_status=0;
        A_out=zeros(N,4);
        reset=0;
    else    % continue homing
        q_des=q_prev + status.*V_mov*dt;   % move legs that have not reached goal
        ready=0;            % homing not finished
        cur_status=0;
        A_out=zeros(N,4);
        reset=0;
    end
end

== matlab function slrt_parker/Force Sensor/Convert from Voltage to Wrench ==
  data: V input; W output; A input; inv_T input
function W = Convert_Function(V,A,inv_T)%A_vec,p)

W = inv_T*A*V;

== matlab function slrt_parker/Trajectory Planner/Quintic Polynomial/trigger detection/MATLAB Function ==
  data: trig input; enable output; trig_history input
function enable= fcn(trig,trig_history)
%#codegen
%%  This func is just to detect a rising trigger
%   Once this rising trigger detected, this manual enable will be locked
%   until mode change
if trig_history==0
    if trig==0
        enable=0;
    else
        enable=1;
    end
else
    enable = 1;
end

== matlab function slrt_parker/Trajectory Planner/Quintic Polynomial/5th Order Polynomial/Embedded MATLAB Function ==
  data: p output; p_des input; p_curr input; tf input; tc input; pdot output; pdotdot output; conf input; confn output; t0 input; t0n output; p0n output; p0 input; enable input; RECORD output
function [p,pdot,pdotdot,confn,t0n,p0n,RECORD] = fifth_order_p(p_des,p_curr,tf,tc,conf,t0,p0,enable)

n = 3;
RECORD = 0;

if enable == 0                  % Configuration space is not used (pdot = 0). 
    p = p_curr;
    pdotdot = zeros(n,1);
    pdot = zeros(n,1);          % However we do want to record the current 
    confn = 0;                  % position in order to be ready as soon 
    t0n = tc;                   % as the enable becomes 1. 
    p0n = p_curr;
else
    if (p_des-p0)'*(p_des-p0) > 0
        if conf == 0                % conf = 0 means that the 5th order poly 
            p0n = p0;               % is not configured for the desired trajectory.
            t0n = tc;               % Therefore, the block is initialized.
            confn = 1;
            pdot = zeros(n,1);
            p = p0;
            pdotdot = zeros(n,1);
        else
            p0n = p0;
            t0n = t0;
            confn = conf;
            % 5th order polynomial
            a0 = p0;
            a4 = -15*(p_des-p0);
            a3 = -2/3 * a4;
            a5 = -2/5 * a4;
            t = tc-t0;
            tau = t/tf;
            if t < tf
                RECORD = 1;
                p = a0 + a3 * tau^3 + a4 * tau^4 + a5 * tau^5;
                pdot = 3*a3*t^2/tf^3 + 4*a4*t^3/tf^4 + 5*a5*t^4/tf^5;
                pdotdot = 6*a3*t/tf^3 + 12*a4*t^2/tf^4 + 20*a5*t^3/tf^5;
            else
                p = p_des;
                pdot = zeros(n,1);
                pdotdot = zeros(n,1);
                p0n = p_des;
            end
        end
    else
        p = p_des;
        pdot = zeros(n,1);
        pdotdot = zeros(n,1);
        confn = 0;
        p0n = p0;
        t0n = t0;
    end
end
%------------------------------------------------------------------------

== matlab function slrt_parker/Force Sensor/Force Stop/MATLAB Function ==
  data: u input; y output
function y = not(u)
%#codegen

y = 1-u;

== matlab function slrt_parker/Trajectory Planner/safety check/false detection ==
  data: pva_cmd input; pva_allowed output; pva_prev input; error_flag output; error_prev input
function [pva_allowed,error_flag] = fcn(pva_cmd,pva_prev,error_prev)
%#codegen
%%  This func is a safety check
%   once the system received some illegal command, the system will be
%   locked for diagnostic purpose
error_flag = 0;
if sum(isnan(pva_cmd))~=0
    error_flag = 1;
end
if sum(isinf(pva_cmd))~=0
    error_flag = 1;
end
if sum(abs(pva_cmd(1:3))>250)~=0 % out of stroke command
    error_flag=1;
end
if error_prev % once faulty, lock down.
    error_flag = 1;
end

if error_flag
    pva_allowed = pva_prev;
else
    pva_allowed = pva_cmd;
end
